simulink model "Week3_Q3"  (R2020b)
settings: Solver=ode45  StartTime=0.0  StopTime=10.0  RelTol=1e-3
InitFcn:
  | g=9.81;
  | I=5;
  | m=75;
  | R=1.25;
  | v0=44;
undefined symbols (not defined in the file): sigbuilder_block
settings Model: Creator=DELL  LastModifiedBy=DELL

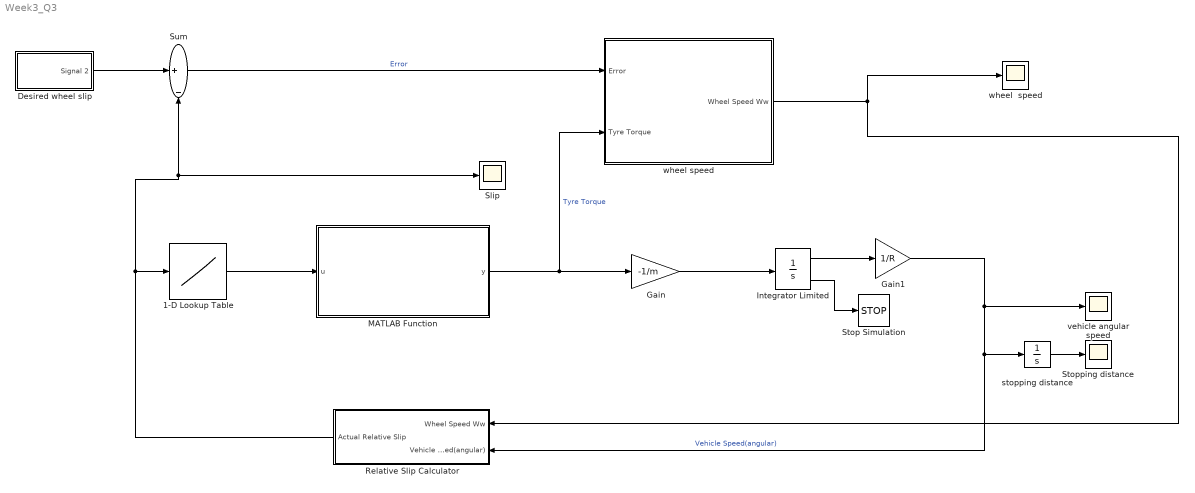
== system Week3_Q3 ==
  1-D Lookup Table : Lookup_n-D  NumberOfTableDimensions=1  BreakpointsForDimension1=[0,0.05,0.1,0.15,0.2,0.25,0.3,0.35,0.4,0.45,0.5,0.55,0.6,0.65,0.7,0.75,0.8,0.85,0.9,0.95,1]  Table=[0,0.4,0.8,0.97,1,0.98,0.96,0.94,0.92,0.9,0.88,0.855,0.83,0.81,0.79,0.77,0.75,0.73,0.72,0.71,0.7]  InternalRulePriority=Speed  RndMeth=Simplest  InputSameDT=on
  Desired wheel slip : Subsystem  Tag=STV Subsys  LoadFcn=sigbuilder_block('load');  StartFcn=sigbuilder_block('start');  StopFcn=sigbuilder_block('stop');  ClipboardFcn=sigbuilder_block('clipboard');  mask(Sigbuilder block){tuvar=[0:10]}
      mask help: Simulink:masks:SigbuilderBlock_MD
      mask init:
      | if ~strcmp(get_param(bdroot(gcbh),'SimulationStatus'),'stopped') tuvar = sigbuilder_block('maskInit'); end
      settings: CopyFcn=sigbuilder_block('copy');  DeleteFcn=sigbuilder_block('delete');  ModelCloseFcn=sigbuilder_block('modelClose');  PreSaveFcn=sigbuilder_block('preSave');  PauseFcn=sigbuilder_block('pause');  ContinueFcn=sigbuilder_block('continue');  NameChangeFcn=sigbuilder_block('namechange');  OpenFcn=sigbuilder_block('open',[437.6 153 550.4 359.25 ]);  CloseFcn=sigbuilder_block('close');
      mask Display: plot(0, 0, 100, 100,[2, 2, 32, 32, 2], [68, 8, 8, 68, 68],[32, 2], [38, 38], [32, 19, 2],[53, 60, 44], [32, 17, 17, 2],[16, 16, 31, 31]);txt = getActiveGroup(gcbh);text(2, 100, txt,'verticalAlignment', 'top');
  Gain : Gain  Gain=-1/m
  Gain1 : Gain  Gain=1/R
  Integrator Limited : Integrator  InitialCondition=v0  LimitOutput=on  UpperSaturationLimit=1000  LowerSaturationLimit=0  ShowSaturationPort=on
  MATLAB Function : MATLAB Function  TreatAsAtomicUnit=on
  Relative Slip Calculator : Subsystem
  Slip : Scope
  Stop Simulation : Stop
  Stopping distance : Scope
  Sum : Sum  Inputs=|+-
  stopping distance : Integrator
  vehicle angular speed : Scope
  wheel  speed : Scope
  wheel speed : Subsystem
  wires:
  Desired wheel slip/1(Signal 2) -> Sum/1
  1-D Lookup Table/1 -> MATLAB Function/1(u)
  Sum/1 -> wheel speed/1(Error)  "Error"
  MATLAB Function/1(y) -> Gain/1, wheel speed/2(Tyre Torque)  "Tyre Torque"
  wheel speed/1(Wheel Speed Ww) -> Relative Slip Calculator/1(Wheel Speed Ww), wheel  speed/1
  Gain/1 -> Integrator Limited/1
  Integrator Limited/1 -> Gain1/1
  Gain1/1 -> Relative Slip Calculator/2(Vehicle Speed(angular)), stopping distance/1, vehicle angular speed/1  "Vehicle Speed(angular)"
  Integrator Limited/2 -> Stop Simulation/1
  stopping distance/1 -> Stopping distance/1
  Relative Slip Calculator/1(Actual Relative Slip) -> 1-D Lookup Table/1, Slip/1, Sum/2

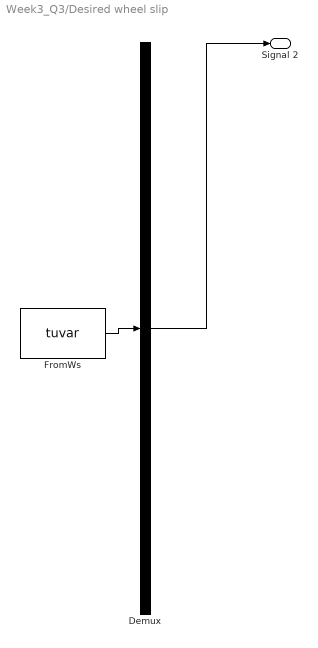
== system Week3_Q3/Desired wheel slip ==
  Demux : Demux  Tag=STV Demux  Outputs=1
      settings: DisplayOption=none
  FromWs : FromWorkspace  Tag=STV FromWs  VariableName=tuvar
      SigBuilderData=|
      | common.afterFinalStr = 'Extrapolate'
      | common.sampleTime = 0
      | dataSet.timeRange = [0 10]
      | dataSet.name = 'Group 1'
      | sbobj.Groups.Name = 'Group 1'
      | sbobj.Groups.Signals.Name = 'Signal 2'
      | sbobj.Groups.Signals.XData = [0 10]
      | sbobj.Groups.Signals.YData = [0.2 0.2]
  Signal 2 : Outport  Tag=STV Outport
  wires:
  FromWs/1 -> Demux/1
  Demux/1 -> Signal 2/1

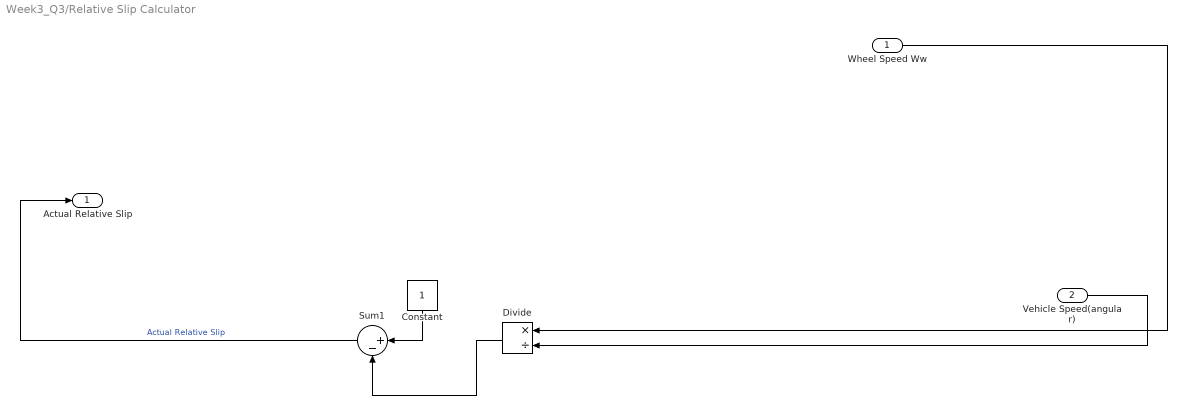
== system Week3_Q3/Relative Slip Calculator ==
  Wheel Speed Ww : Inport
  Vehicle Speed(angular) : Inport  Port=2
  Constant : Constant
  Divide : Product  Inputs=*/
  Sum1 : Sum  Inputs=|+-
  Actual Relative Slip : Outport
  wires:
  Constant/1 -> Sum1/1
  Vehicle Speed(angular)/1 -> Divide/2
  Divide/1 -> Sum1/2
  Wheel Speed Ww/1 -> Divide/1
  Sum1/1 -> Actual Relative Slip/1  "Actual Relative Slip"

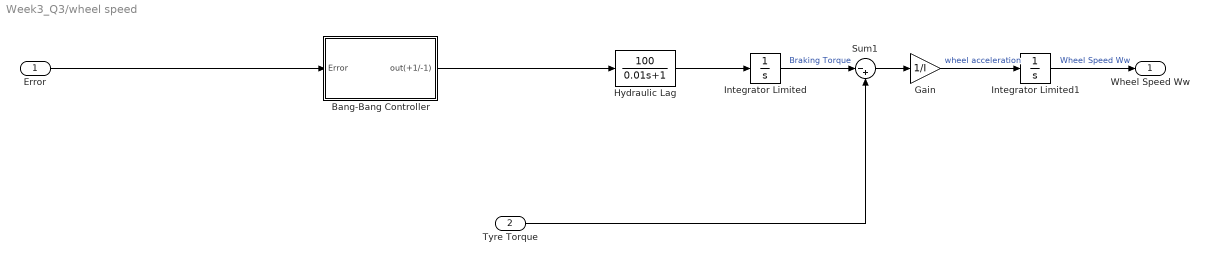
== system Week3_Q3/wheel speed ==
  Error : Inport
  Tyre Torque : Inport  Port=2
  Bang-Bang Controller : Subsystem
  Gain : Gain  Gain=1/I
  Hydraulic Lag : TransferFcn  Numerator=[100]  Denominator=[0.01 1]
  Integrator Limited : Integrator  LimitOutput=on  UpperSaturationLimit=1000  LowerSaturationLimit=0
  Integrator Limited1 : Integrator  InitialCondition=v0/R  LimitOutput=on  UpperSaturationLimit=1000  LowerSaturationLimit=0
  Sum1 : Sum  Inputs=|-+
  Wheel Speed Ww : Outport
  wires:
  Hydraulic Lag/1 -> Integrator Limited/1
  Sum1/1 -> Gain/1
  Error/1 -> Bang-Bang Controller/1(Error)
  Gain/1 -> Integrator Limited1/1  "wheel acceleration"
  Integrator Limited/1 -> Sum1/1  "Braking Torque"
  Bang-Bang Controller/1(out(+1/-1)) -> Hydraulic Lag/1
  Tyre Torque/1 -> Sum1/2
  Integrator Limited1/1 -> Wheel Speed Ww/1  "Wheel Speed Ww"

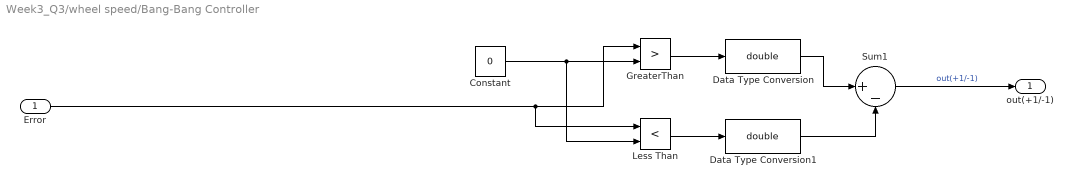
== system Week3_Q3/wheel speed/Bang-Bang Controller ==
  Error : Inport
  Constant : Constant  Value=0
  Data Type Conversion : DataTypeConversion  OutDataTypeStr=double  RndMeth=Zero
  Data Type Conversion1 : DataTypeConversion  OutDataTypeStr=double  RndMeth=Zero
  GreaterThan : RelationalOperator  Operator=>  OutDataTypeStr=boolean  RndMeth=Simplest
  Less Than : RelationalOperator  Operator=<  OutDataTypeStr=boolean  RndMeth=Simplest
  Sum1 : Sum  Inputs=|+-
  out(+1/-1) : Outport
  wires:
  Error/1 -> Less Than/1, GreaterThan/1
  Constant/1 -> Less Than/2, GreaterThan/2
  Data Type Conversion1/1 -> Sum1/2
  Less Than/1 -> Data Type Conversion1/1
  Data Type Conversion/1 -> Sum1/1
  Sum1/1 -> out(+1/-1)/1  "out(+1/-1)"
  GreaterThan/1 -> Data Type Conversion/1

== matlab function Week3_Q3/MATLAB Function ==
  data: u input; y output
function y = fcn(u)

m=75;
g=9.81;
R=1.25;
y=m*g*R*u/4;
